simulink model "mpc_block"  (R2025b)
settings: Solver=VariableStepAuto  StartTime=0.0  StopTime=10.0  RelTol=1e-3
InitFcn:
  | m = 1;
  | v_0 = [0; 0; 0];
  | q_0 = [1; 0; 0; 0];
  | omega_0 = [0; 0; 0];
  | T_0 = [0; 0; 9.81 * m];
  | u_0 = [0; 0; 0];
  | 
  | ts = 0.05;
  | 
  | [A, B, C, D, DX] = computePlantMats(v_0, q_0, omega_0, T_0, u_0);
  | PlantSS = ss(A, B, C, D, ts);
  | mpc_obj = mpc(PlantSS, ts);
  | 
  | elems(1) = Simulink.BusElement;
  | elems(1).Name = 'A';
  | elems(1).Dimensions = size(A);
  | elems(2) = Simulink.BusElement;
  | elems(2).Name = 'B';
  | elems(2).Dimensions = size(B);
  | elems(3) = Simulink.BusElement;
  | elems(3).Name = 'C';
  | elems(3).Dimensions = size(C);
  | elems(4) = Simulink.BusElement;
  | elems(4).Name = 'D';
  | elems(4).Dimensions = size(D);
  | elems(5) = Simulink.BusElement;
  | elems(5).Name = 'U';
  | elems(5).Dimensions = [3 1];
  | elems(6) = Simulink.BusElement;
  | elems(6).Name = 'Y';
  | elems(6).Dimensions = [16 1];
  | elems(7) = Simulink.BusElement;
  | elems(7).Name = 'X';
  | elems(7).Dimensions = [16 1];
  | elems(8) = Simulink.BusElement;
  | elems(8).Name = 'DX';
  | elems(8).Dimensions = [16 1];
  | 
  | StateSpaceBus = Simulink.Bus;
  | StateSpaceBus.Elements = elems;
  | 
  | set_param(bdroot, 'BusNameAdapt', 'WarnAndRepair');
  | 
  | mpc_obj.PredictionHorizon = 10;
  | mpc_obj.ControlHorizon = 3;
  | mpc_obj.Weights.OV = [10 10 10,  1 1 1,  ...
  |     5 5 5 5,  1 1 1,  0.1 0.1 0.1];
  | mpc_obj.Weights.MV = [0.1, 0.1, 0.1];
model workspace (MAT data in the model file):
  Object = Simulink.LookupTable
  Object.Table = Simulink.lookuptable.Table
  Object.Table.Dimensions = [0 0]
  Object.Table.DataType = 'auto'
  Object.Table.FieldName = 'Table'
  Object.Breakpoints = Simulink.lookuptable.Breakpoint
  Object.Breakpoints.TunableSizeName = 'N1'
  Object.Breakpoints.TunableSizeValue = -1
  Object.Breakpoints.Dimensions = [0 0]
  Object.Breakpoints.DataType = 'auto'
  Object.Breakpoints.FieldName = 'BP1'
  Object.AllowMultipleInstancesOfTypeToHaveDifferentTableBreakpointSizes = 0
  Object.SupportTunableSize = 0
  Object.StructTypeInfo = Simulink.lookuptable.StructTypeInfo
  Object.StructTypeInfo.DataScope = 'Auto'
  Var = 0
libraries: mpclib x1
settings Model: Creator=user  LastModifiedBy=user
settings DebuggingCC: BusObjectLabelMismatch=none

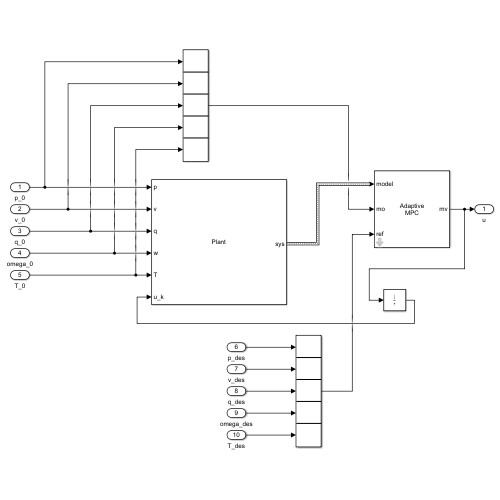
[thumbnail: Simulink's stored preview of the top-level diagram]
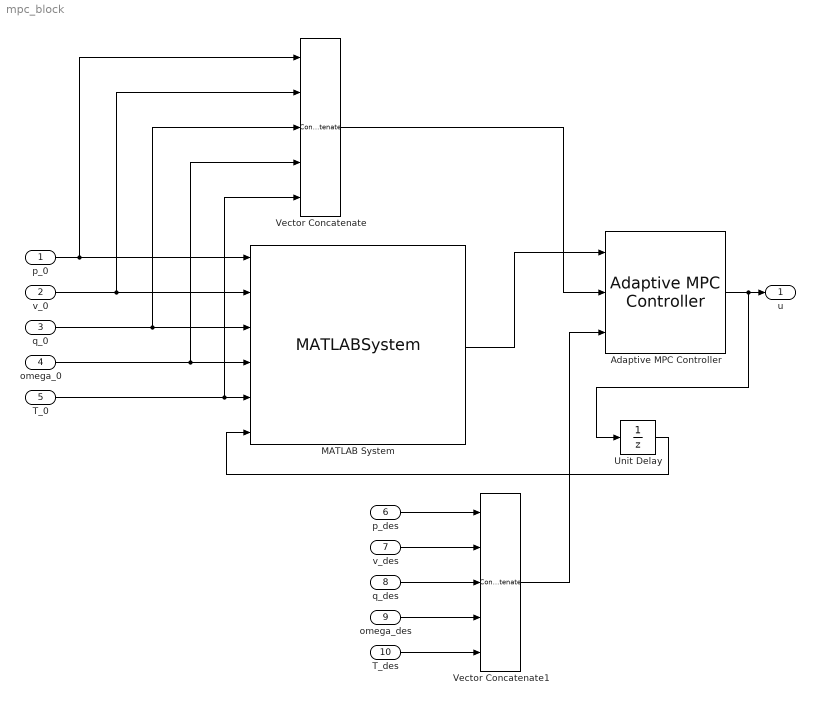
== system mpc_block ==
  p_0 : Inport  PortDimensions=3
  v_0 : Inport  Port=2  PortDimensions=3
  q_0 : Inport  Port=3  PortDimensions=4
  omega_0 : Inport  Port=4  PortDimensions=3
  T_0 : Inport  Port=5  PortDimensions=3
  p_des : Inport  Port=6  PortDimensions=3
  v_des : Inport  Port=7  PortDimensions=3
  q_des : Inport  Port=8  PortDimensions=4
  omega_des : Inport  Port=9  PortDimensions=3
  T_des : Inport  Port=10  PortDimensions=3
  Adaptive MPC Controller : mpclib/Adaptive MPC Controller  SCDEnableBlockLinearizationSpecification=on  mpcobj=mpc_obj  enable_value=0  updateMPCinCallerWorkspace=on  md_inport=off  mv_inport=off  uref_inport=off  return_cost=off  return_mvseq=off  return_qpstatus=off  return_xseq=off  return_state=off  return_ovseq=off  state_inport=off  isltv_plant=off  umin_inport=off  umax_inport=off  ymin_inport=off  ymax_inport=off  cc_inport=off  ywt_inport=off  uwt_inport=off  duwt_inport=off  rhoeps_inport=off  pm_inport=off  MaximumP=10  HorizonChoice=FixedHorizon  BlockDataType=double  SampleTimeInherited=off  switch_inport=off
  MATLAB System : MATLABSystem  System=Plant  SimulateUsing=Code generation
      mask Type: Plant
  Unit Delay : UnitDelay  SampleTime=-1  HasFrameUpgradeWarning=on
  Vector Concatenate : Concatenate  NumInputs=5
  Vector Concatenate1 : Concatenate  NumInputs=5
  u : Outport
  wires:
  p_0/1 -> Vector Concatenate/1, MATLAB System/1
  p_des/1 -> Vector Concatenate1/1
  v_des/1 -> Vector Concatenate1/2
  omega_des/1 -> Vector Concatenate1/4
  omega_0/1 -> Vector Concatenate/4, MATLAB System/4
  T_0/1 -> Vector Concatenate/5, MATLAB System/5
  v_0/1 -> Vector Concatenate/2, MATLAB System/2
  q_0/1 -> Vector Concatenate/3, MATLAB System/3
  Vector Concatenate/1 -> Adaptive MPC Controller/2
  q_des/1 -> Vector Concatenate1/3
  T_des/1 -> Vector Concatenate1/5
  Vector Concatenate1/1 -> Adaptive MPC Controller/3
  Adaptive MPC Controller/1 -> Unit Delay/1, u/1
  MATLAB System/1 -> Adaptive MPC Controller/1
  Unit Delay/1 -> MATLAB System/6
